simulink model "temp_4"  (R2020b)
settings: Solver=VariableStepAuto  StartTime=0.0  StopTime=10.0  RelTol=1e-3
settings Model: Creator=Jonathan van Zyl  LastModifiedBy=Jonathan van Zyl

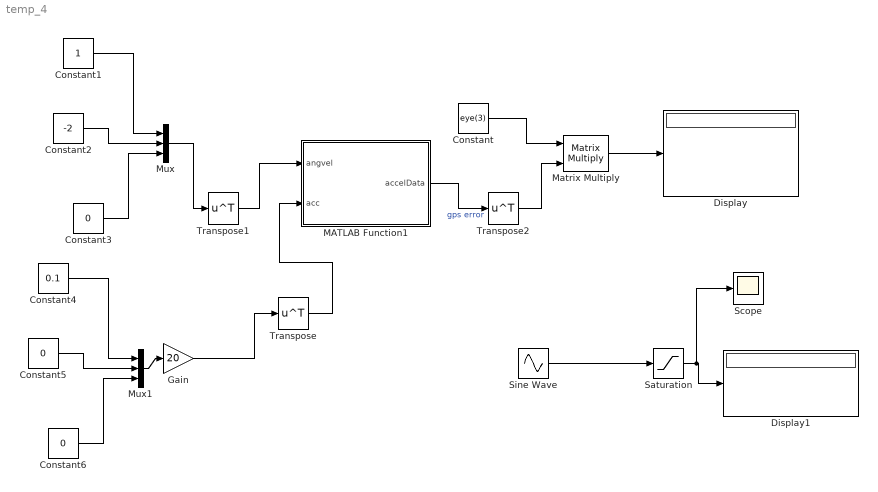
== system temp_4 ==
  Constant : Constant  Value=eye(3)
  Constant1 : Constant
  Constant2 : Constant  Value=-2
  Constant3 : Constant  Value=0
  Constant4 : Constant  Value=0.1
  Constant5 : Constant  Value=0
  Constant6 : Constant  Value=0
  Display : Display
  Display1 : Display
  Gain : Gain  Gain=20
  MATLAB Function1 : MATLAB Function  TreatAsAtomicUnit=on
  Matrix Multiply : Product  Multiplication=Matrix(*)
  Mux : Mux  Inputs=3
  Mux1 : Mux  Inputs=3
  Saturation : Saturate
  Scope : Scope
  Sine Wave : Sin  SampleTime=0
  Transpose : Math  Operator=transpose  SaturateOnIntegerOverflow=on
  Transpose1 : Math  Operator=transpose  SaturateOnIntegerOverflow=on
  Transpose2 : Math  Operator=transpose  SaturateOnIntegerOverflow=on
  wires:
  MATLAB Function1/1(accelData) -> Transpose2/1  "gps error"
  Constant1/1 -> Mux/1
  Constant2/1 -> Mux/2
  Constant3/1 -> Mux/3
  Constant5/1 -> Mux1/2
  Constant4/1 -> Mux1/1
  Constant6/1 -> Mux1/3
  Mux1/1 -> Gain/1
  Mux/1 -> Transpose1/1
  Gain/1 -> Transpose/1
  Transpose/1 -> MATLAB Function1/2(acc)
  Transpose1/1 -> MATLAB Function1/1(angvel)
  Constant/1 -> Matrix Multiply/1
  Matrix Multiply/1 -> Display/1
  Transpose2/1 -> Matrix Multiply/2
  Sine Wave/1 -> Saturation/1
  Saturation/1 -> Scope/1, Display1/1

== matlab function temp_4/MATLAB Function1 ==
  data: angvel input; accelData output; acc input
function accelData = accelerometer(angvel, acc)

    %
    % Create gyroscope sensor object
    params = accelparams 
    
    % Parameters for simulated signal
    N = 1;       % Number of samples
    Fs = 100;       % Sampling rate
    Fc = 0.25;      % Sinusoidal frequency
    
    
    % Create arrays
    t = (0:(1/Fs):((N-1)/Fs)).';
    acc = acc;          %Input accelerations
    orient = quaternion.ones(N, 1);
    angvel = angvel;
    
    % Generate acceleration data
    imu = imuSensor('SampleRate', Fs, 'Accelerometer', params);
    imu.Accelerometer.MeasurementRange = 1000;   % Maximum acceleration accelerometer can measure
    imu.Accelerometer.Resolution = 1/Fs;           % Step size of digital measurements
    
    % Biases
    imu.Accelerometer.BiasInstability = 7.5 / 1000 * 9.81;
    imu.Accelerometer.NoiseDensity = 150 / 1000 / 1000 * 9.81; 
    imu.Accelerometer.TemperatureBias = 50 / 1000 / 1000 * 9.81;
    
  
    
    accelData = imu(acc, angvel, orient);
    
    accelData(:,3) = accelData(:,3) - 9.81

    accelData(:,1) = accelData(:,1) * -1
    accelData(:,2) = accelData(:,2) * -1
    accelData(:,3) = accelData(:,3) * -1

end
